simulink model "simBoth"  (R2020a)
settings: Solver=ode3  StartTime=0.0  StopTime=simPrm.tEnd  FixedStep=simPrm.dt  MaxStep=1/30  RelTol=1e-3  EnableMultiTasking=on
values from neighbouring files (symbols this model uses):
  Ac = [ 0    0        1     0 ... (first row only)    [setupBoth.m]
  Ad = [0    0           1     0 ... (first row only)    [setupBoth.m]
  Bc = [0;0;Mat.B31;Mat.B41]    [setupBoth.m]
  Bd = [0;0;Mat.Bd31;0]    [setupBoth.m]
  Cc = [1 0 0 0 ... (first row only)    [setupBoth.m]
  Cd = [1 0 0 0 ... (first row only)    [setupBoth.m]
  Dc = [0;0;0;0]    [setupBoth.m]
  Dd = [0;0;0;0]    [setupBoth.m]
  Kp = Omega_n^2/(Calc.d/Calc.a1)    [setupBoth.m]
undefined symbols (not defined in the file or in its folder): Input
settings Model: Creator=ggparker  LastModifiedBy=vmali
settings DataIOCC: LimitDataPoints=on
settings OptimizationCC: LifeSpan=inf
settings DebuggingCC: AllowSymbolicDim=off  SFUnexpectedBacktrackingDiag=warning  SFNoUnconditionalDefaultTransitionDiag=warning  SFExecutionAtInitializationDiag=none  ArithmeticOperatorsInVariantConditions=warning
settings SFSimCC: SimUseLocalCustomCode=off  CustomCodeUndefinedFunction=UseInterfaceOnly
settings RTWCC: RTWUseLocalCustomCode=off
settings CodeAppCC: StateflowObjectComments=on
settings GRTTargetCC: TargetLangStandard=C89/C90 (ANSI)
settings ConfigComp: CovMetricSettings=dw  CovHtmlReporting=on  CovSaveCumulativeToWorkspaceVar=on  CovSaveSingleToWorkspaceVar=on  CovExternalEMLEnable=off  CovSFcnEnable=off
settings SimscapeCC: SimscapeNominalValues="[{\"value\":\"10\",\"unit\":\"V\"},{\"value\":\"1\",\"unit\":\"A\"},{\"value\":\"10\",\"unit\":\"N*m\"},{\"value\":\"10\",\"unit\":\"bar\"},{\"value\":\"100\",\"unit\":\"kJ/kg\"},{\"value\":\"1\",\"unit\":\"kW\"},{\"value\":\"300\",\"unit\":\"K\"},{\"value\":\"100\",\"unit\":\"cm^3/s\"},{\"value\":\"1\",\"unit\":\"kN\"},{\"value\":\"1\",\"unit\":\"g/cm^3\"},{\"value\":\"1\",\"unit\":\"l\"},{\"value\":\"1\",\"unit\":\"cm^2\"},{\"value\":\"60\",\"unit\":\"Hz\"}]"  SimscapeLogType=all  SimscapeLogToSDI=on  SimscapeLogDataHistory=10000
settings ConfigurationSet: Description=SimMechanics 2G

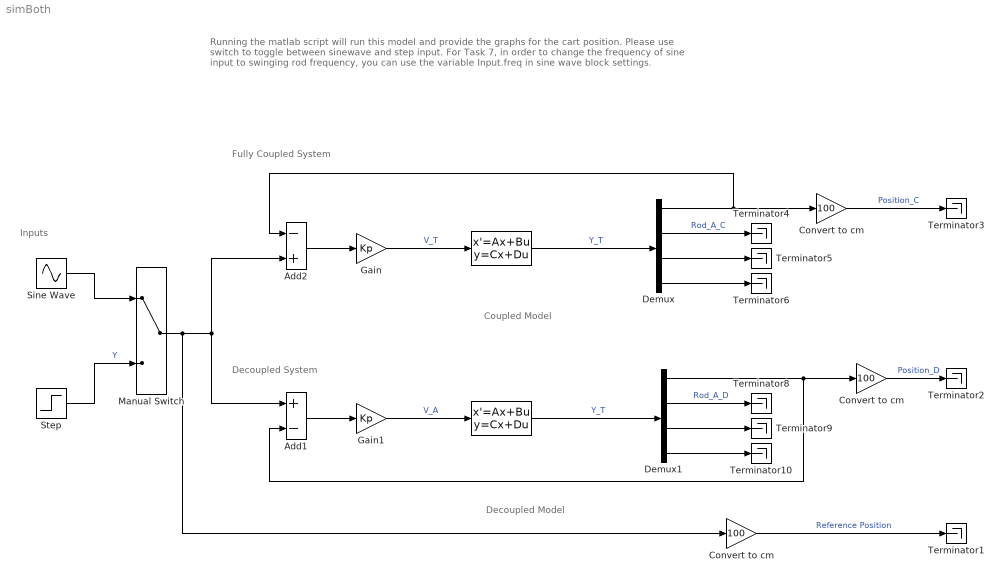
== system simBoth ==
  note: Running the matlab script will run this model and provide the graphs for the cart position.
      | Please use switch to toggle between sinewave and step input.
      | For Task 7, in order to change the frequency of sine input to swinging rod frequency,
      | you can use the variable Input.freq in sine wave block settings.
  note: Coupled Model
  note: Decoupled System
  note: Fully Coupled System
  note: Inputs
  note: Decoupled Model
  " " : StateSpace  A=Ac  B=Bc  C=Cc  D=Dc  InitialCondition=[0;0;0;0]
  "  " : StateSpace  A=Ad  B=Bd  C=Cd  D=Dd  InitialCondition=[0;0;0;0]
  Add1 : Sum  Inputs=+-
  Add2 : Sum  Inputs=-+
  Convert to cm : Gain  Gain=100
  "Convert to cm " : Gain  Gain=100
  "Convert to cm  " : Gain  Gain=100
  Demux : Demux
  Demux1 : Demux
  Gain : Gain  Gain=Kp
  Gain1 : Gain  Gain=Kp
  Manual Switch : ManualSwitch
  Sine Wave : Sin  Amplitude=Input.Ref  Frequency=1.0  SampleTime=0
  Step : Step  After=Input.Ref  SampleTime=0
  Terminator{1..6,8..10} (9 alike) : Terminator
  wires:
  " "/1 -> Demux/1  "Y_T"
  Sine Wave/1 -> Manual Switch/1
  Step/1 -> Manual Switch/2  "Y"
  Add1/1 -> Gain1/1
  Add2/1 -> Gain/1
  Gain/1 -> " "/1  "V_T"
  Gain1/1 -> "  "/1  "V_A"
  Demux/2 -> Terminator4/1  "Rod_A_C"
  Demux/3 -> Terminator5/1
  Demux/4 -> Terminator6/1
  Demux1/4 -> Terminator10/1
  Demux1/3 -> Terminator9/1
  Demux1/1 -> "Convert to cm "/1, Add1/2
  "  "/1 -> Demux1/1  "Y_T"
  Demux1/2 -> Terminator8/1  "Rod_A_D"
  Demux/1 -> "Convert to cm  "/1, Add2/1
  Manual Switch/1 -> Convert to cm/1, Add1/1, Add2/2
  Convert to cm/1 -> Terminator1/1  "Reference Position"
  "Convert to cm "/1 -> Terminator2/1  "Position_D"
  "Convert to cm  "/1 -> Terminator3/1  "Position_C"
